simulink model "custom_model"  (R2017a)
settings: Solver=ode15s  StartTime=0.0  StopTime=4e5  RelTol=1e-3
settings Model: Creator=Vera  LastModifiedBy=Vera
settings DataIOCC: LimitDataPoints=on  SaveFormat=Array
settings OptimizationCC: LifeSpan=inf
settings ModelReferenceCC: ModelReferenceNumInstancesAllowed=Single  PropagateSignalLabelsOutOfModel=off

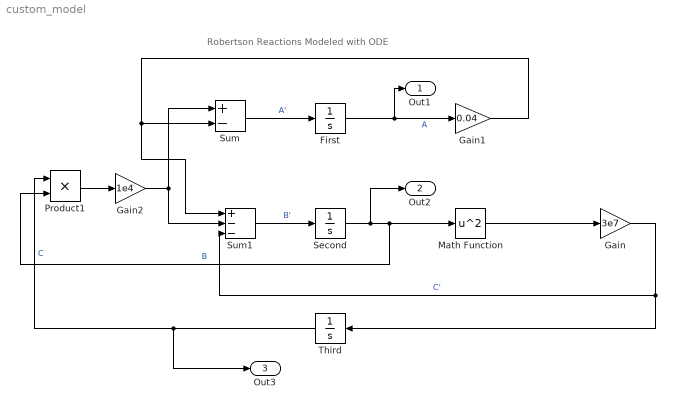
== system custom_model ==
  note: Robertson Reactions Modeled with ODE
  First : Integrator  InitialCondition=1
  Gain : Gain  Gain=3e7
  Gain1 : Gain  Gain=0.04
  Gain2 : Gain  Gain=1e4
  Math Function : Math  Operator=square  SaturateOnIntegerOverflow=on
  Product1 : Product
  Second : Integrator
  Sum : Sum  Inputs=+-
  Sum1 : Sum  Inputs=+--
  Third : Integrator
  Out1 : Outport
  Out2 : Outport  Port=2
  Out3 : Outport  Port=3
  wires:
  Sum/1 -> First/1  "A'"
  First/1 -> Out1/1, Gain1/1  "A"
  Sum1/1 -> Second/1  "B'"
  Second/1 -> Out2/1, Product1/2, Math Function/1  "B"
  Math Function/1 -> Gain/1
  Gain1/1 -> Sum1/1, Sum/2
  Product1/1 -> Gain2/1
  Third/1 -> Out3/1, Product1/1  "C"
  Gain/1 -> Sum1/3, Third/1  "C'"
  Gain2/1 -> Sum/1, Sum1/2
